simulink model "main"  (R2021a)
settings: Solver=ode113  StartTime=0.0  StopTime=100  RelTol=1e-13  AbsTol=1e-14
values from neighbouring files (symbols this model uses):
  Earth =     [workspace.mat]
  Sensors =     [workspace.mat]
  Spacecraft =     [workspace.mat]
undefined symbols (not defined in the file or in its folder): initCond
libraries: aerolibutil x48, vrlib x31, dspsrcs4 x29, simulink x10, SADlibrary x8, commfilt2 x3, sharedtransform x3, dspfdesign x3, sharedutil x2, sharedTrackingLibrary x2, dspmathops x1
(part 3 of 3)

== matlab function main/Subsystem1/Sun sensor reading4/Subsystem/MATLAB Function ==
  data: theta input; q output
function q = aboutBoresightRotation(theta)

q = [cos(theta/2) 0 0 sin(theta/2)];

== matlab function main/Subsystem1/Sun sensor reading4/Subsystem/MATLAB Function2 ==
  data: theta input; q output size=[1 4]; e input
function q = crossBoresightRotation(theta,e)

q = [cos(theta/2) sin(theta/2)*[e(1) e(2)] 0];

== matlab function main/Subsystem1/Sun sensor reading5/Subsystem/MATLAB Function ==
  data: theta input; q output
function q = aboutBoresightRotation(theta)

q = [cos(theta/2) 0 0 sin(theta/2)];

== matlab function main/Subsystem1/Sun sensor reading5/Subsystem/MATLAB Function2 ==
  data: theta input; q output size=[1 4]; e input
function q = crossBoresightRotation(theta,e)

q = [cos(theta/2) sin(theta/2)*[e(1) e(2)] 0];

== matlab function main/Subsystem1/Sun sensor reading/Subsystem/MATLAB Function2 ==
  data: theta input; q output size=[1 4]; e input
function q = crossBoresightRotation(theta,e)

q = [cos(theta/2) sin(theta/2)*[e(1) e(2)] 0];

== matlab function main/Subsystem1/MATLAB Function1 ==
  data: s output size=[2 1]; s1 input; q_SB1 input; s2 input; q_SB2 input; s3 input; q_SB3 input; s4 input; q_SB4 input; s5 input; q_SB5 input; s6 input; sensAtt output; q_SB6 input
function [s,sensAtt] =  getSunSensorReading(s1,q_SB1,s2,q_SB2,s3,q_SB3,s4,q_SB4,s5,q_SB5,s6,q_SB6)
[~,i] = min([sum(s1.^2) sum(s2.^2) sum(s3.^2) sum(s4.^2) sum(s5.^2) sum(s6.^2)]);
switch i
    case 1
        s = s1;
        sensAtt = q_SB1;
    case 2
        s = s2;
        sensAtt = q_SB2;
    case 3
        s = s3;
        sensAtt = q_SB3;
    case 4
        s = s4;
        sensAtt = q_SB4;
    case 5
        s = s5;
        sensAtt = q_SB5;
    case 6
        s = s6;
        sensAtt = q_SB6;
    otherwise
        error("Errore");
end

== matlab function main/Solve Whabba's problem/MATLAB Function4 ==
  data: start_SF input; S output; V output; in2 input
function [S,V] = fromSensorScreenToBodyFrame(start_SF,in2)
nStar = numel(start_SF)/2;

S = zeros(3,nStar);
V = zeros(3,nStar);

% From star sensor frame to body frame
q_SB = in2(1:4);
A_SB = [           1-2*q_SB(3)^2-2*q_SB(4)^2  2*q_SB(2)*q_SB(3)+2*q_SB(1)*q_SB(4) -2*q_SB(1)*q_SB(3)+2*q_SB(2)*q_SB(4) ;...
         2*q_SB(2)*q_SB(3)-2*q_SB(1)*q_SB(4)            1-2*q_SB(2)^2-2*q_SB(4)^2  2*q_SB(1)*q_SB(2)+2*q_SB(3)*q_SB(4) ;...
         2*q_SB(1)*q_SB(3)+2*q_SB(2)*q_SB(4) -2*q_SB(1)*q_SB(2)+2*q_SB(3)*q_SB(4)              1-2*q_SB(2)^2-2*q_SB(3)^2 ];

% Star in ECI
j = 1;
for i=5:3:(3*nStar+4)
    V(:,j) = in2(i:i+2);
    j = j+1;
end

% Star in body frame
j = 1;
for i=1:2:(2*nStar)
    S(:,j) = [tan(start_SF(i)) tan(start_SF(i+1)) 1]';
    S(:,j) = S(:,j) / norm(S(:,j));
    S(:,j) = A_SB*S(:,j);
    j = j+1;
end

== matlab function main/Comparison/MATLAB Function ==
  data: q input; e output
function e = fcn(q)
e = sqrt(q(2)^2+q(3)^2+q(4)^2) * 180 / pi * 2;

== matlab function main/Comparison/MATLAB Function1 ==
  data: q input; e output
function e = fcn(q)
e = sqrt(q(2)^2+q(3)^2+q(4)^2) * 180 / pi * 2;

== matlab function main/Solve Whabba's problem/MATLAB Function ==
  data: B input; K output
function K = fromBtoK(B)
S = B+B';
sigma = trace(B);
Z = [B(2,3)-B(3,2) B(3,1)-B(1,3) B(1,2)-B(2,1)]';

K = [sigma             Z';...
         Z S-sigma*eye(3)];
